simulink model "dc_motor"  (R2020b)
settings: Solver=VariableStepAuto  StartTime=0.0  StopTime=30  RelTol=1e-3
model workspace: external: MATLAB File C:\Users\matti\OneDrive\Documents\4th Year\ELEC-391\pendulum-control\src\constants.m (data not in the file)
values from neighbouring files (symbols this model uses):
  K_b = 22.09592    [constants.m]
  K_m = 0.0452    [constants.m]
  Ze_den = [7.46e-7 7.25]    [constants.m]
  Ze_num = [1]    [constants.m]
  Zm_den = [(3.9774e-6 + 8.82e-7) 0.000805]    [constants.m]
  Zm_num = [1]    [constants.m]
settings Model: OrderedModelArguments=off  Creator=matti  LastModifiedBy=matti

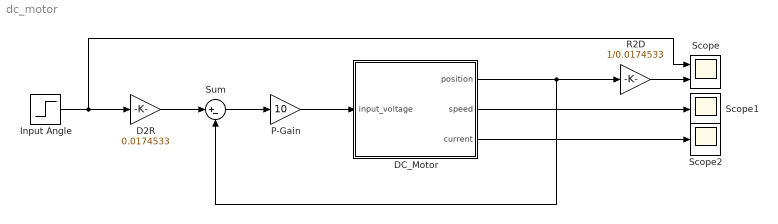
== system dc_motor ==
  D2R : Gain  Gain=0.0174533
  "DC_Motor " : Subsystem
  Input Angle : Step  After=45  SampleTime=0
  P-Gain : Gain  Gain=10
  R2D : Gain  Gain=1/0.0174533
  Scope : Scope  NumInputPorts=2
  Scope1 : Scope
  Scope2 : Scope
  Sum : Sum  Inputs=|+-
  wires:
  "DC_Motor "/1(position) -> R2D/1, Sum/2
  "DC_Motor "/2(speed) -> Scope1/1
  P-Gain/1 -> "DC_Motor "/1(input_voltage)
  Sum/1 -> P-Gain/1
  Input Angle/1 -> Scope/1, D2R/1
  D2R/1 -> Sum/1
  R2D/1 -> Scope/2
  "DC_Motor "/3(current) -> Scope2/1

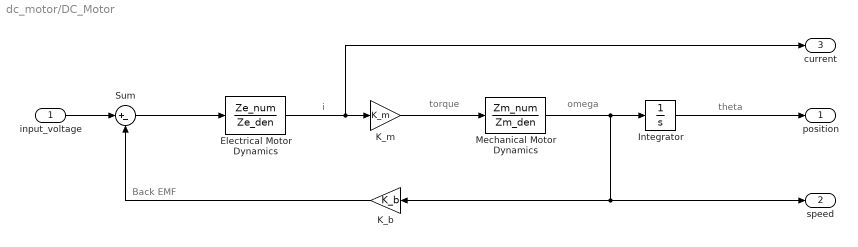
== system dc_motor/DC_Motor  ==
  note: theta
  note: omega
  note: torque
  note: i
  note: Back EMF
  input_voltage : Inport
  Electrical Motor Dynamics : TransferFcn  Numerator=Ze_num  Denominator=Ze_den
  Integrator : Integrator
  K_b : Gain  Gain=K_b
  K_m : Gain  Gain=K_m
  Mechanical Motor Dynamics : TransferFcn  Numerator=Zm_num  Denominator=Zm_den
  Sum : Sum  Inputs=|+-
  position : Outport
  speed : Outport  Port=2
  current : Outport  Port=3
  wires:
  Mechanical Motor Dynamics/1 -> speed/1, K_b/1, Integrator/1
  K_b/1 -> Sum/2
  Integrator/1 -> position/1
  Electrical Motor Dynamics/1 -> current/1, K_m/1
  K_m/1 -> Mechanical Motor Dynamics/1
  Sum/1 -> Electrical Motor Dynamics/1
  input_voltage/1 -> Sum/1
